simulink model "bergman_model"  (R2024b)
settings: Solver=ode4  StartTime=0  StopTime=600  FixedStep=0.1  RelTol=1e-3
undefined symbols (not defined in the file): out
libraries: simulink x2, slpidlib x1, fuzblock x1
settings Model: Creator=luca1  LastModifiedBy=luca1

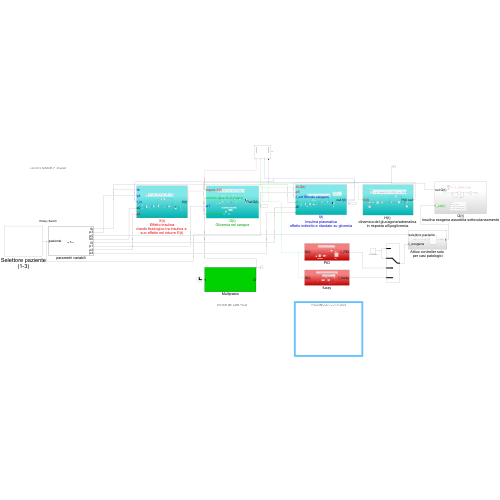
[thumbnail: Simulink's stored preview of the top-level diagram]
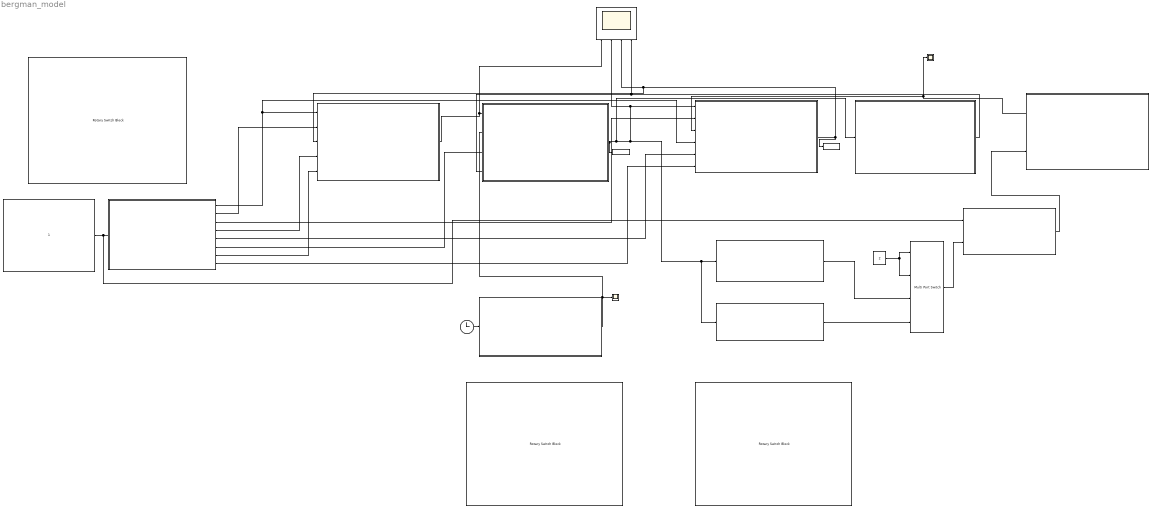
== system bergman_model ==
  Attiva controller solo per casi patologici : Subsystem
  Clock : Clock
  "G(t) Glicemia nel sangue " : Subsystem
  H(t) dinamica del glucagone/adrenalina in risposta all’ipoglicemia. : Subsystem
  I(t) Insulina plasmatica effetto indiretto e ritardato su glicemia : Subsystem
  INSULINA ESOGENA : Constant  Value=2
  Multipasto : MATLAB Function  TreatAsAtomicUnit=on
  Multiport Switch : MultiPortSwitch  DataPortOrder=Zero-based contiguous  zeroidx=on  SaturateOnIntegerOverflow=off  InputSameDT=off
  PID : Subsystem
  Q(t) Insulina esogena assorbita sottocutaneamente : Subsystem
      settings: PortSchema="{\"entries\":[{\"content\":{\"sides\":[{\"content\":{\"connectorIds\":[\"Out1\",\"In1\"]},\"type\":\"ConnectorPlacement.EquallySpacedRectSide\",\"uuid\":\"1f913c37-221a-4650-b88f-17f5a316c6cf\"},{\"content\":{\"side\":\"RIGHT\"},\"type\":\"ConnectorPlacement.EquallySpacedRectSide\",\"uuid\":\"e18204c5-ef25-406d-920f-cf79c2c01384\"},{\"content\":{\"side\":\"TOP\"},\"type\":\"ConnectorPlacement.EquallySpacedRectSide\",\"uuid\":\"310f9809-d6a5-4270-bb3b-6c96e71083e8\"}]},\"type\":\"ConnectorPlacement.EquallySpacedConnector\",\"uuid\":\"4efd81b8-14ef-4bdd-919a-dabc5923124a\"}],\"packageUris\":[\"http://schema.mathworks.com/mf0/Connector/R2020b\"],\"version\":\"1.0\"}"
  Rotary Switch : RotarySwitchBlock
      settings: Values={{'Sano', 'Tipo 1', 'Tipo 2'}, [1 2 3]}
  Rotary Switch1 : RotarySwitchBlock
      settings: Values={{'Light', 'Medium', 'High'}, [0.1 0.15 0.2]}
  Rotary Switch3 : RotarySwitchBlock
      settings: Values={{'Off', 'PID', 'Fuzzy'}, [0 1 2]}
  Scope : Scope  NumInputPorts=4
      settings: Description=Grafici
  Scope1 : Scope
  Scope2 : Scope
  Selettore paziente (1-3) : Constant
  To Workspace2 : ToWorkspace  VariableName=G  SaveFormat=Timeseries  SampleTime=-1
  To Workspace3 : ToWorkspace  VariableName=I  SaveFormat=Timeseries  SampleTime=-1
  X(t) Effetto insulina ritardo fisiologico tra insulina e suo effetto nel ridurre G(t) : Subsystem
  fuzzy : Subsystem
  parametri variabili : MATLAB Function  TreatAsAtomicUnit=on
  wires:
  X(t) Effetto insulina ritardo fisiologico tra insulina e suo effetto nel ridurre G(t)/1(X(t)) -> "G(t) Glicemia nel sangue "/1(inport: X(t)), Scope/1
  I(t) Insulina plasmatica effetto indiretto e ritardato su glicemia/1(out I(t)) -> To Workspace3/1, X(t) Effetto insulina ritardo fisiologico tra insulina e suo effetto nel ridurre G(t)/3(I_in), Scope/3
  Selettore paziente (1-3)/1 -> Attiva controller solo per casi patologici/1(selettore paziente), parametri variabili/1(paziente)
  parametri variabili/1(Ib) -> X(t) Effetto insulina ritardo fisiologico tra insulina e suo effetto nel ridurre G(t)/1(Ib), I(t) Insulina plasmatica effetto indiretto e ritardato su glicemia/4(Ib)
  parametri variabili/2(p3) -> X(t) Effetto insulina ritardo fisiologico tra insulina e suo effetto nel ridurre G(t)/2(p3)
  parametri variabili/3(p5) -> I(t) Insulina plasmatica effetto indiretto e ritardato su glicemia/2(p5)
  Multipasto/1(D) -> "G(t) Glicemia nel sangue "/2(stimolo glicemico (pasto)), Scope2/1
  "G(t) Glicemia nel sangue "/1(Out G(t)) -> H(t) dinamica del glucagone/adrenalina in risposta all’ipoglicemia./1(G(t)), fuzzy/1(G(t)), PID/1(G(t)), I(t) Insulina plasmatica effetto indiretto e ritardato su glicemia/1(In G(t)), Scope/2, To Workspace2/1
  parametri variabili/4(X0) -> X(t) Effetto insulina ritardo fisiologico tra insulina e suo effetto nel ridurre G(t)/4(x0)
  parametri variabili/5(I0) -> I(t) Insulina plasmatica effetto indiretto e ritardato su glicemia/5(I0)
  parametri variabili/6(p1) -> "G(t) Glicemia nel sangue "/3(p1)
  INSULINA ESOGENA/1 -> Multiport Switch/2, Multiport Switch/1
  fuzzy/1(I_fuzzy) -> Multiport Switch/4
  PID/1(I_PID) -> Multiport Switch/3
  parametri variabili/7(p2) -> X(t) Effetto insulina ritardo fisiologico tra insulina e suo effetto nel ridurre G(t)/5(p2)
  parametri variabili/8(p4) -> I(t) Insulina plasmatica effetto indiretto e ritardato su glicemia/6(p4)
  Q(t) Insulina esogena assorbita sottocutaneamente/1(out Q(t)) -> Scope1/1, I(t) Insulina plasmatica effetto indiretto e ritardato su glicemia/3(I_ext Stimolo esogeno)
  Multiport Switch/1 -> Attiva controller solo per casi patologici/2(I_esogena)
  Attiva controller solo per casi patologici/1(Out1) -> Q(t) Insulina esogena assorbita sottocutaneamente/1(I_ext(t))
  Clock/1 -> Multipasto/1(t)
  H(t) dinamica del glucagone/adrenalina in risposta all’ipoglicemia./1(H(t) out) -> Scope/4, "G(t) Glicemia nel sangue "/4(H(T) inport)

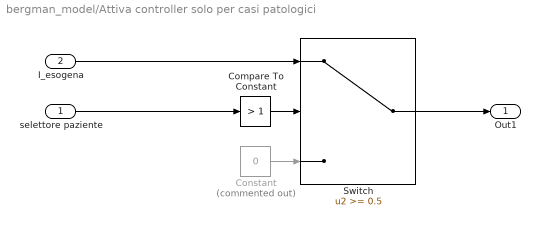
== system bergman_model/Attiva controller solo per casi patologici ==
  selettore paziente : Inport
  I_esogena : Inport  Port=2
  Compare To Constant : simulink/Logic and Bit Operations/Compare To Constant  relop=>  const=1  OutDataTypeStr=boolean
  Constant : Constant  Commented=on  Value=0
  Switch : Switch  Threshold=0.5  SaturateOnIntegerOverflow=off  InputSameDT=off
  Out1 : Outport
  wires:
  Compare To Constant/1 -> Switch/2
  Constant/1 -> Switch/3
  selettore paziente/1 -> Compare To Constant/1
  I_esogena/1 -> Switch/1
  Switch/1 -> Out1/1

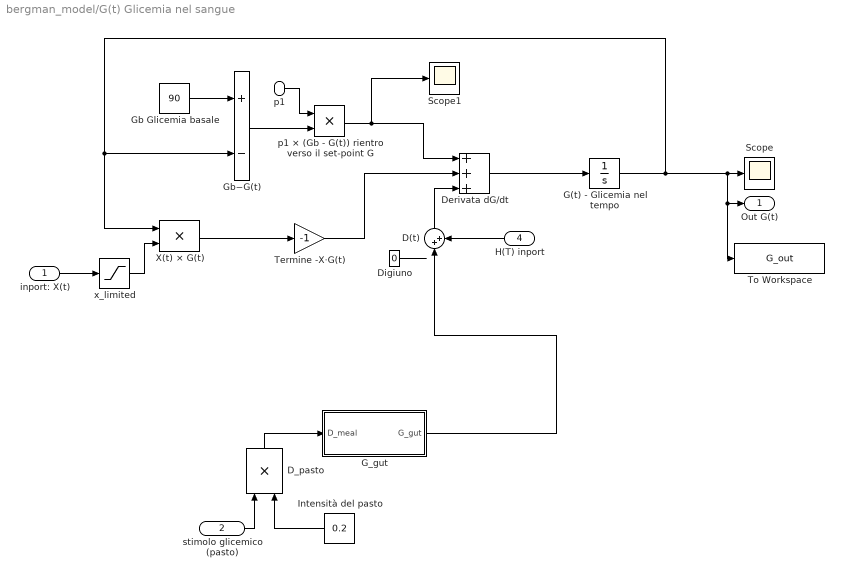
== system bergman_model/G(t) Glicemia nel sangue  ==
  inport: X(t) : Inport
  stimolo glicemico (pasto) : Inport  Port=2
  p1 : Inport  Port=3
  H(T) inport : Inport  Port=4
  D(t) : Sum  Inputs=|++
  D_pasto : Product
  "Derivata dG/dt " : Sum  Inputs=+++
  Digiuno : Constant  Value=0
  G(t) - Glicemia nel tempo : Integrator  InitialCondition=100
  G_gut : Subsystem
  Gb Glicemia basale : Constant  Value=90
  Gb−G(t) : Sum  Inputs=+-
  Intensità del pasto : Constant  Value=0.2
  Scope : Scope
  Scope1 : Scope
  Termine -X·G(t) : Gain  Gain=-1
  To Workspace : ToWorkspace  VariableName=G_out  SaveFormat=Structure With Time  SampleTime=-1
  X(t) × G(t) : Product
  p1 × (Gb - G(t)) rientro verso il set-point G : Product
  x_limited : Saturate  UpperLimit=inf  LowerLimit=0
  Out G(t) : Outport
  wires:
  Gb Glicemia basale/1 -> Gb−G(t)/1
  G(t) - Glicemia nel tempo/1 -> Scope/1, To Workspace/1, Out G(t)/1, Gb−G(t)/2, X(t) × G(t)/1
  Gb−G(t)/1 -> p1 × (Gb - G(t)) rientro verso il set-point G/2
  X(t) × G(t)/1 -> Termine -X·G(t)/1
  Termine -X·G(t)/1 -> "Derivata dG/dt "/2
  p1 × (Gb - G(t)) rientro verso il set-point G/1 -> Scope1/1, "Derivata dG/dt "/1
  "Derivata dG/dt "/1 -> G(t) - Glicemia nel tempo/1
  stimolo glicemico (pasto)/1 -> D_pasto/1
  Intensità del pasto/1 -> D_pasto/2
  inport: X(t)/1 -> x_limited/1
  x_limited/1 -> X(t) × G(t)/2
  Digiuno/1 -> ?
  p1/1 -> p1 × (Gb - G(t)) rientro verso il set-point G/1
  D(t)/1 -> "Derivata dG/dt "/3
  H(T) inport/1 -> D(t)/2
  G_gut/1(G_gut) -> D(t)/1
  D_pasto/1 -> G_gut/1(D_meal)

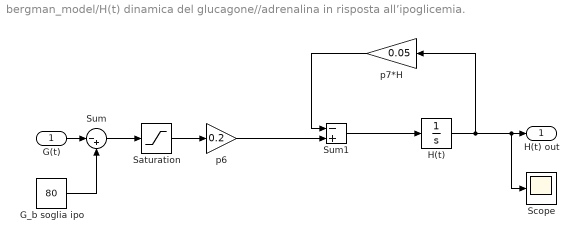
== system bergman_model/H(t) dinamica del glucagone//adrenalina in risposta all’ipoglicemia. ==
  G(t) : Inport
  G_b soglia ipo : Constant  Value=80
  H(t) : Integrator
  Saturation : Saturate  UpperLimit=inf  LowerLimit=0
  Scope : Scope
  Sum : Sum  Inputs=|-+
  Sum1 : Sum  Inputs=-+
  p6 : Gain  Gain=0.2
  p7*H : Gain  Gain=0.05
  H(t) out : Outport
  wires:
  H(t)/1 -> p7*H/1, Scope/1, H(t) out/1
  p7*H/1 -> Sum1/1
  G(t)/1 -> Sum/1
  G_b soglia ipo/1 -> Sum/2
  Sum/1 -> Saturation/1
  Saturation/1 -> p6/1
  p6/1 -> Sum1/2
  Sum1/1 -> H(t)/1

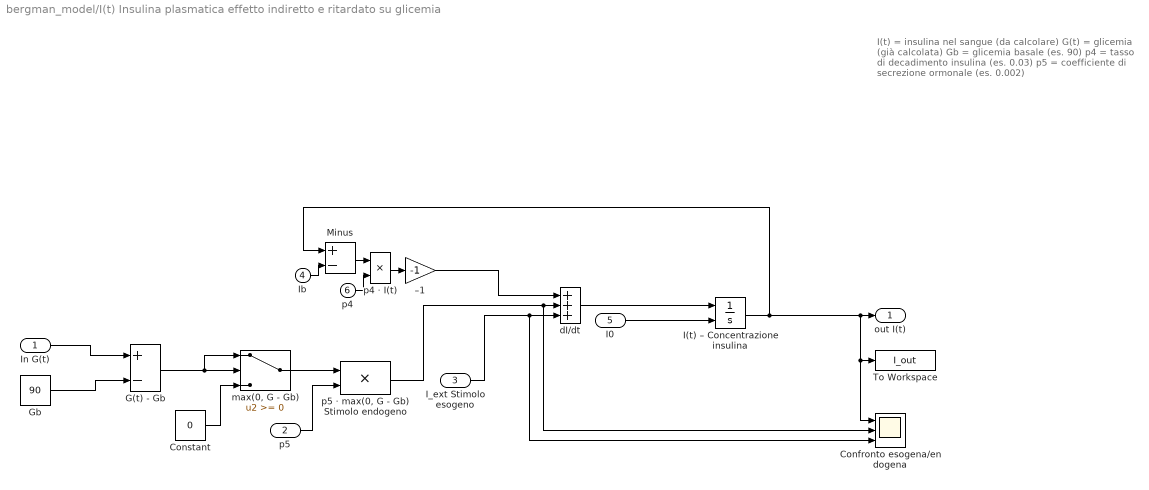
== system bergman_model/I(t) Insulina plasmatica effetto indiretto e ritardato su glicemia ==
  note: I(t) = insulina nel sangue (da calcolare)
      | G(t) = glicemia (già calcolata)
      | Gb = glicemia basale (es. 90)
      | p4 = tasso di decadimento insulina (es. 0.03)
      | p5 = coefficiente di secrezione ormonale (es. 0.002)
  In G(t) : Inport
  p5 : Inport  Port=2
  I_ext Stimolo esogeno : Inport  Port=3
  Ib : Inport  Port=4
  I0 : Inport  Port=5
  p4 : Inport  Port=6
  Confronto esogena/endogena : Scope  NumInputPorts=3
  Constant : Constant  Value=0
  G(t) - Gb : Sum  Inputs=+-
  Gb : Constant  Value=90
  "I(t) – Concentrazione insulina " : Integrator  InitialConditionSource=external  InitialCondition=out.I0
  Minus : Sum  Inputs=+-
  To Workspace : ToWorkspace  VariableName=I_out  SaveFormat=Structure With Time  SampleTime=-1
  dI/dt : Sum  Inputs=+++
  "max(0, G - Gb)" : Switch  SaturateOnIntegerOverflow=off  InputSameDT=off
  p4 · I(t) : Product
  "p5 · max(0, G - Gb) Stimolo endogeno" : Product
  –1 : Gain  Gain=-1
  out I(t) : Outport
  wires:
  "I(t) – Concentrazione insulina "/1 -> Confronto esogena/endogena/1, To Workspace/1, out I(t)/1, Minus/1
  In G(t)/1 -> G(t) - Gb/1
  Gb/1 -> G(t) - Gb/2
  G(t) - Gb/1 -> "max(0, G - Gb)"/1, "max(0, G - Gb)"/2
  Constant/1 -> "max(0, G - Gb)"/3
  "max(0, G - Gb)"/1 -> "p5 · max(0, G - Gb) Stimolo endogeno"/1
  –1/1 -> dI/dt/1
  "p5 · max(0, G - Gb) Stimolo endogeno"/1 -> Confronto esogena/endogena/2, dI/dt/2
  dI/dt/1 -> "I(t) – Concentrazione insulina "/1
  p5/1 -> "p5 · max(0, G - Gb) Stimolo endogeno"/2
  I_ext Stimolo esogeno/1 -> Confronto esogena/endogena/3, dI/dt/3
  Minus/1 -> p4 · I(t)/1
  Ib/1 -> Minus/2
  I0/1 -> "I(t) – Concentrazione insulina "/2
  p4/1 -> p4 · I(t)/2
  p4 · I(t)/1 -> –1/1

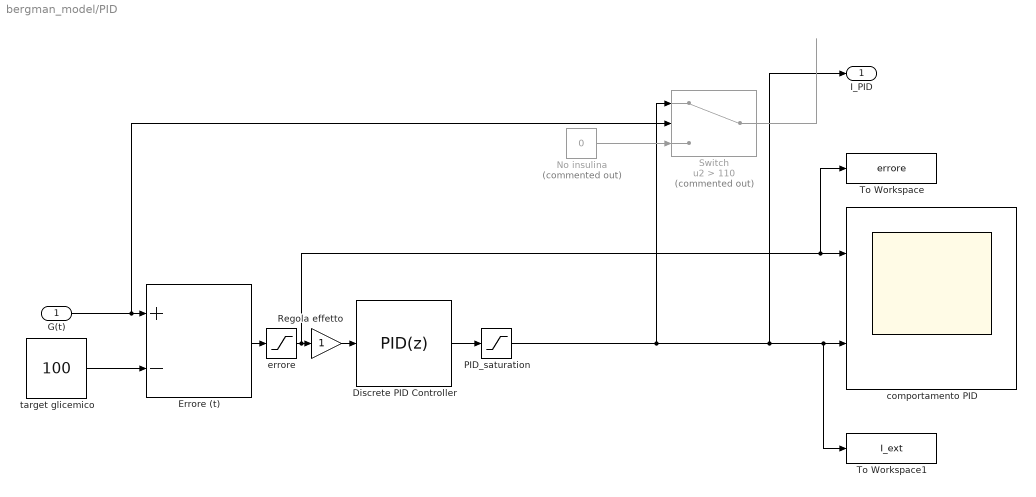
== system bergman_model/PID ==
  G(t) : Inport
  Discrete PID Controller : slpidlib/PID Controller  Controller=PID  Form=Parallel  TimeDomain=Discrete-time  UseExternalTs=off  SampleTime=-1  IntegratorMethod=Forward Euler  FilterMethod=Forward Euler  ControllerParametersSource=internal  P=1  I=0.01  UseKiTs=off  D=0.05  UseExternalDerivativeSource=off  N=10  UseFilter=on  TunerSelectOption=Transfer Function Based (PID Tuner App)  InitialConditionSource=internal  InitialConditionForIntegrator=0  InitialConditionForFilter=0  DifferentiatorICPrevScaledInput=0  ExternalReset=none  TrackingMode=off  Kt=1  LimitOutput=on  SatLimitsSource=internal  UpperSaturationLimit=30  LowerSaturationLimit=0  LinearizeAsGain=off  AntiWindupMode=clamping  Kb=1  LimitIntegrator=on  UpperIntegratorSaturationLimit=30  LowerIntegratorSaturationLimit=0  POutMin=[]  POutMax=[]  IOutMin=[]  IOutMax=[]  DOutMin=[]  DOutMax=[]  NOutMin=[]  NOutMax=[]  SumOutMin=[]  SumOutMax=[]  SaturationOutMin=[]  SaturationOutMax=[]  PParamMin=[]  PParamMax=[]  IParamMin=[]  IParamMax=[]  DParamMin=[]  DParamMax=[]  NParamMin=[]  NParamMax=[]  KbParamMin=[]  KbParamMax=[]  KtParamMin=[]  KtParamMax=[]  KbOutMin=[]  KbOutMax=[]  KtOutMin=[]  KtOutMax=[]  IntegratorOutMin=[]  IntegratorOutMax=[]  FilterOutMin=[]  FilterOutMax=[]  SumI1OutMin=[]  SumI1OutMax=[]  SumI2OutMin=[]  SumI2OutMax=[]  SumI3OutMin=[]  SumI3OutMax=[]  SumI4OutMin=[]  SumI4OutMax=[]  SumDOutMin=[]  SumDOutMax=[]  DifferentiatorOutMin=[]  DifferentiatorOutMax=[]  FilterDiffOutCoefMin=[]  FilterDiffOutCoefMax=[]  ReciprocalOutMin=[]  ReciprocalOutMax=[]  SumDenOutMin=[]  SumDenOutMax=[]  SumNumOutMin=[]  SumNumOutMax=[]  DivideOutMin=[]  DivideOutMax=[]  UdiffTsProdOutMin=[]  UdiffTsProdOutMax=[]  NTsProdOutMin=[]  NTsProdOutMax=[]  UintegralTsProdOutMin=[]  UintegralTsProdOutMax=[]  UngainTsProdOutMin=[]  UngainTsProdOutMax=[]  ClampingZeroOutDataTypeStr=Inherit: Inherit via back propagation  ClampingZeroOutMin=[]  ClampingZeroOutMax=[]  FilterDenConstantOutDataTypeStr=Inherit: Inherit via back propagation  FilterDenConstantOutMin=[]  FilterDenConstantOutMax=[]  PCopyOutDataTypeStr=Inherit: Inherit via back propagation  PCopyOutMin=[]  PCopyOutMax=[]  NCopyOutDataTypeStr=Inherit: Inherit via back propagation  NCopyOutMin=[]  NCopyOutMax=[]  IntegratorContinuousStateAttributes=''  IntegratorStateMustResolveToSignalObject=off  IntegratorRTWStateStorageClass=Auto  FilterContinuousStateAttributes=''  FilterStateMustResolveToSignalObject=off  FilterRTWStateStorageClass=Auto  ParallelPVariant=InternalParameters  IdealPVariant=Disabled  IVariant=InternalParameters  DVariant=InternalParameters  IntegratorVariant=Discrete  SatVariant=Enabled  AWVariant=DiscClampingParallel  PCopyVariant=Disabled  TRVariant=Disabled  FdbkBlocksVariant=Forward  IdealPFdbkVariant=Disabled  SatFdbkVariant=Disabled  DerivativeFilterVariant=ForwardEulerFilter  NVariant=InternalParameters  NCopyVariant=Disabled  FilterICVariant=InternalICsFilter  IntegratorICVariant=InternalICs  ExternalResetVariant=Disabled  TRSumVariant=Passthrough  SumFdbkVariant=Disabled  SumVariant=Sum_PID  TsampFilterVariant=InternalTs  TsampNgainVariant=Passthrough  TsampIntegralVariant=Disabled_SignalSpec  ExternalSaturationOutDataTypeStr=Inherit: Same as second input  DerivativeSourceVariant=ErrorSignal  PreIntVariant=InternalPreInt
      settings: LibrarySourceBlock=simulink/Discrete/Discrete PID Controller
  Errore (t) : Sum  Inputs=+-
  No insulina : Constant  Commented=on  Value=0
  PID_saturation : Saturate  UpperLimit=30  LowerLimit=0
  Regola effetto : Gain
  Switch : Switch  Commented=on  Criteria=u2 > Threshold  Threshold=110  SaturateOnIntegerOverflow=off  InputSameDT=off
  To Workspace : ToWorkspace  VariableName=errore  SaveFormat=Timeseries  SampleTime=-1
  To Workspace1 : ToWorkspace  VariableName=I_ext  SaveFormat=Timeseries  SampleTime=-1
  comportamento PID : Scope  NumInputPorts=2
  errore : Saturate  UpperLimit=5  LowerLimit=-5
  target glicemico : Constant  Value=100
  I_PID : Outport
  wires:
  Regola effetto/1 -> Discrete PID Controller/1
  Errore (t)/1 -> errore/1
  PID_saturation/1 -> I_PID/1, comportamento PID/2, To Workspace1/1, Switch/1
  No insulina/1 -> Switch/3
  Discrete PID Controller/1 -> PID_saturation/1
  errore/1 -> comportamento PID/1, To Workspace/1, Regola effetto/1
  target glicemico/1 -> Errore (t)/2
  G(t)/1 -> Switch/2, Errore (t)/1
  Switch/1 -> ?

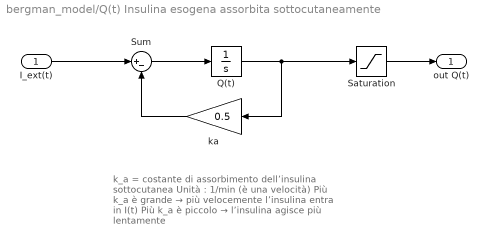
== system bergman_model/Q(t) Insulina esogena assorbita sottocutaneamente ==
  note: k_a = costante di assorbimento dell’insulina sottocutanea
      | Unità : 1/min (è una velocità)
      | Più k_a è grande → più velocemente l’insulina entra in I(t)
      | Più k_a è piccolo → l’insulina agisce più lentamente
  I_ext(t) : Inport
  Q(t) : Integrator
  Saturation : Saturate  UpperLimit=6  LowerLimit=-inf
  Sum : Sum  Inputs=|+-
  ka : Gain  Gain=0.5
  out Q(t) : Outport
  wires:
  Q(t)/1 -> Saturation/1, ka/1
  I_ext(t)/1 -> Sum/1
  ka/1 -> Sum/2
  Sum/1 -> Q(t)/1
  Saturation/1 -> out Q(t)/1

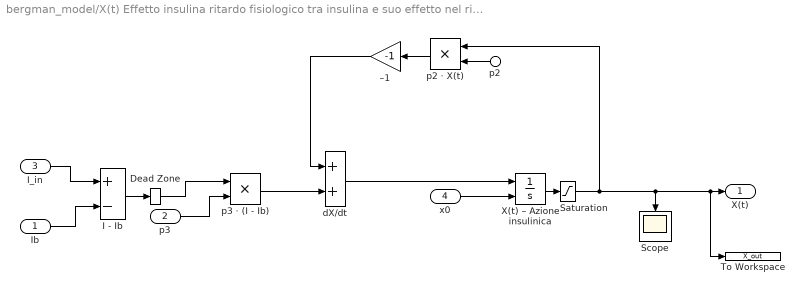
== system bergman_model/X(t) Effetto insulina ritardo fisiologico tra insulina e suo effetto nel ridurre G(t) ==
  Ib : Inport
  p3 : Inport  Port=2
  I_in : Inport  Port=3
  x0 : Inport  Port=4
  p2 : Inport  Port=5
  Dead Zone : DeadZone
  I - Ib : Sum  Inputs=+-
  Saturation : Saturate  UpperLimit=inf  LowerLimit=0
  Scope : Scope
  To Workspace : ToWorkspace  VariableName=X_out  SaveFormat=Structure With Time  SampleTime=-1
  X(t) – Azione insulinica : Integrator  InitialConditionSource=external  InitialCondition=out.x0
  dX/dt : Sum
  p2 · X(t) : Product
  p3 · (I - Ib) : Product
  –1 : Gain  Gain=-1
  X(t) : Outport
  wires:
  I_in/1 -> I - Ib/1
  Ib/1 -> I - Ib/2
  –1/1 -> dX/dt/1
  p3 · (I - Ib)/1 -> dX/dt/2
  dX/dt/1 -> X(t) – Azione insulinica/1
  Dead Zone/1 -> p3 · (I - Ib)/1
  p3/1 -> p3 · (I - Ib)/2
  X(t) – Azione insulinica/1 -> Saturation/1
  I - Ib/1 -> Dead Zone/1
  x0/1 -> X(t) – Azione insulinica/2
  p2/1 -> p2 · X(t)/2
  p2 · X(t)/1 -> –1/1
  Saturation/1 -> To Workspace/1, X(t)/1, Scope/1, p2 · X(t)/1

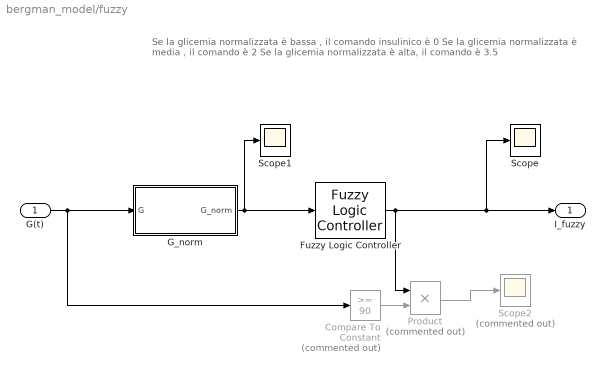
== system bergman_model/fuzzy ==
  note: Se la glicemia normalizzata è bassa , il comando insulinico è 0
      | Se la glicemia normalizzata è media , il comando è 2
      | Se la glicemia normalizzata è alta, il comando è 3.5
  G(t) : Inport
  Compare To Constant : simulink/Logic and Bit Operations/Compare To Constant  Commented=on  relop=>=  const=90  OutDataTypeStr=boolean
  Fuzzy Logic Controller : fuzblock/Fuzzy Logic  Controller  FIS='fuzzy_diabete.fis'  OutputSampleNumber=101  DataType=double  FuzzifiedInputs=off  RuleFiringStrengths=off  RuleOutputs=off  AggregatedOutputs=off  SimulateUsing=Interpreted execution  OutOfRangeInputValueMessage=warning  NoRuleFiredMessage=warning  EmptyOutputFuzzySetMessage=warning
  G_norm : MATLAB Function  TreatAsAtomicUnit=on
  Product : Product  Commented=on
  Scope : Scope
  Scope1 : Scope
  Scope2 : Scope  Commented=on
  I_fuzzy : Outport
  wires:
  G(t)/1 -> Compare To Constant/1, G_norm/1(G)
  G_norm/1(G_norm) -> Fuzzy Logic Controller/1, Scope1/1
  Compare To Constant/1 -> Product/2
  Fuzzy Logic Controller/1 -> Product/1, I_fuzzy/1, Scope/1
  Product/1 -> Scope2/1

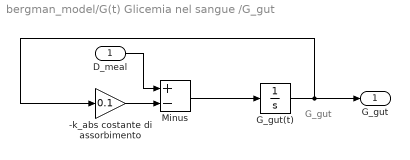
== system bergman_model/G(t) Glicemia nel sangue /G_gut ==
  note: G_gut
  D_meal : Inport
  -k_abs costante di assorbimento : Gain  Gain=0.1
  G_gut(t) : Integrator
  Minus : Sum  Inputs=+-
  G_gut : Outport
  wires:
  D_meal/1 -> Minus/1
  G_gut(t)/1 -> -k_abs costante di assorbimento/1, G_gut/1
  -k_abs costante di assorbimento/1 -> Minus/2
  Minus/1 -> G_gut(t)/1

== matlab function bergman_model/Multipasto ==
  data: t input; D output
function D = Multipasto(t)

% Parametri dei 3 pasti
A1 = 2;      t1 = 60;        sigma1 = 20;   % Colazione
A2 = 2.5;    t2 = 240;       sigma2 = 25;   % Pranzo
A3 = 2;      t3 = 420;       sigma3 = 20;   % Cena

% Curve gaussiane
curva1 = A1 * exp(-(t - t1)^2/(2*sigma1^2));
curva2 = A2 * exp(-(t - t2)^2/(2*sigma2^2));
curva3 = A3 * exp(-(t - t3)^2/(2*sigma3^2));

% Output totale
D = curva1 + curva2 + curva3;

== matlab function bergman_model/parametri variabili ==
  data: paziente input; Ib output; p3 output; p5 output; X0 output; I0 output; p1 output; p2 output; p4 output
function [Ib, p3, p5, X0, I0, p1, p2,p4] = ParametriPaziente(paziente)
    switch paziente
        case 1  % sano
            Ib = 15;
            p1 = 0.04;
            p2 = 0.025;
            p3 = 0.00013;
            p4 = 0.03;
            p5 = 0.005;
            X0 = 0.025;
            I0 = 18;
        case 2  % tipo 1
            Ib = 0;
            p1 = 0;
            p2 = 0.7;
            p3 = 0.00013;
            p4 = 0.03;
            p5 = 0;
            X0 = 0; 
            I0 = 0;
        case 3  % tipo 2
            Ib = 15;
            p1 = 0.02;
            p2 = 0.1;
            p3 = 0.00002;
            p4 = 0.03;
            p5 = 0.002;
            X0 = 0.015;
            I0 = 16;
        otherwise
            % Default safe values (not used, just to avoid errors)
            Ib = 0; p1 = 0; p2 = 0; p3 = 0; p4 = 0; p5 = 0; X0 = 0; I0 = 0;

    end
    % Ib_global = Ib;
    % p3_global = p3;
    % p5_global = p5;
end

== matlab function bergman_model/fuzzy/G_norm ==
  data: G input; G_norm output
function G_norm = fcn(G)

G_norm = (G - 80) / 30;
G_norm = min(max(G_norm, 0), 2);  
G_norm = max(min((G - 80)/30, 1.99), 0.01);
